simulink model "motor_cc_ej5"  (R2024a)
settings: Solver=VariableStepAuto  StartTime=0.0  StopTime=50  RelTol=1e-3
settings Model: Creator=jorge  LastModifiedBy=jorge

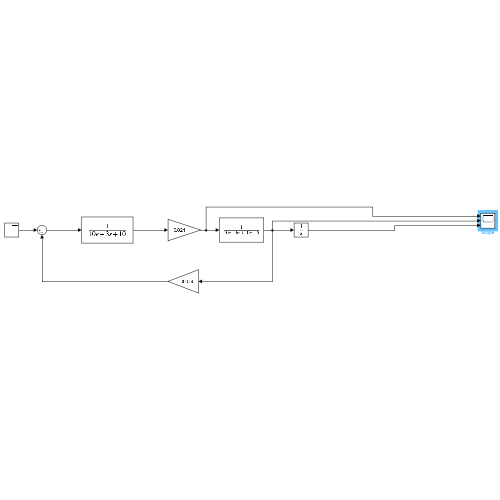
[thumbnail: Simulink's stored preview of the top-level diagram]
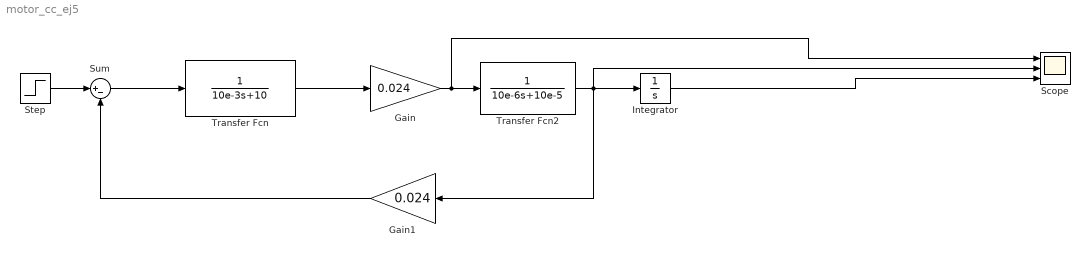
== system motor_cc_ej5 ==
  Gain : Gain  Gain=0.024
  Gain1 : Gain  Gain=0.024
  Integrator : Integrator
  Scope : Scope  NumInputPorts=3
  Step : Step  Time=0  After=24  SampleTime=0.001
  Sum : Sum  Inputs=|+-
  Transfer Fcn : TransferFcn  Denominator=[10e-3 10]
  Transfer Fcn2 : TransferFcn  Denominator=[10e-6 10e-5]
  wires:
  Transfer Fcn2/1 -> Scope/2, Gain1/1, Integrator/1
  Sum/1 -> Transfer Fcn/1
  Transfer Fcn/1 -> Gain/1
  Gain/1 -> Scope/1, Transfer Fcn2/1
  Gain1/1 -> Sum/2
  Step/1 -> Sum/1
  Integrator/1 -> Scope/3
